simulink model "tvc_sim"  (R2019b)
settings: Solver=FixedStepAuto  StartTime=0.0  StopTime=3  FixedStep=0.001  RelTol=1e-3
values from neighbouring files (symbols this model uses):
  Ft = 300    [dynamics_gui.m]    (also in tvc.m)
  I = 3.5    [dynamics_gui.m]    (also in tvc.m)
  Kd = 60    [dynamics_gui.m]    (also in tvc.m = 5)
  Ki = 0    [dynamics_gui.m]    (also in tvc.m)
  Kp = 20    [dynamics_gui.m]    (also in tvc.m = 40)
  theta_0 = 15    [tvc.m]
  theta_des = 0    [tvc.m]
  theta_max = 30    [tvc.m]
  x_cm = 1.2    [dynamics_gui.m]    (also in tvc.m)
settings Model: Creator=seant  LastModifiedBy=SPak
settings DataIOCC: ReturnWorkspaceOutputs=off
settings DebuggingCC: ArithmeticOperatorsInVariantConditions=warning
settings SFSimCC: SimUseLocalCustomCode=off  CustomCodeUndefinedFunction=UseInterfaceOnly
settings RTWCC: RTWUseLocalCustomCode=off

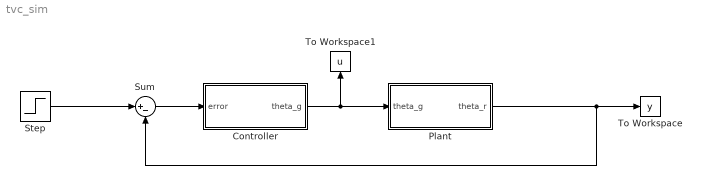
== system tvc_sim ==
  "Controller " : Subsystem
  "Plant " : Subsystem
  Step : Step  Time=0  After=theta_des  SampleTime=0
  Sum : Sum  Inputs=|+-
  To Workspace : ToWorkspace  VariableName=y  SaveFormat=Timeseries  SampleTime=-1
  To Workspace1 : ToWorkspace  VariableName=u  SaveFormat=Timeseries  SampleTime=-1
  wires:
  Step/1 -> Sum/1
  "Controller "/1(theta_g) -> "Plant "/1("theta_g "), To Workspace1/1
  Sum/1 -> "Controller "/1(error)
  "Plant "/1(theta_r) -> Sum/2, To Workspace/1

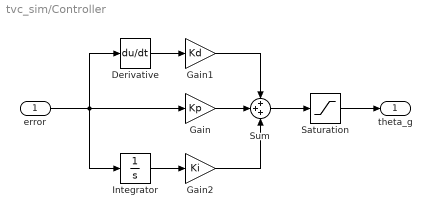
== system tvc_sim/Controller  ==
  error : Inport
  Derivative : Derivative
  Gain : Gain  Gain=Kp
  Gain1 : Gain  Gain=Kd
  Gain2 : Gain  Gain=Ki
  Integrator : Integrator
  Saturation : Saturate  UpperLimit=deg2rad(theta_max)  LowerLimit=-deg2rad(theta_max)
  Sum : Sum  Inputs=+++
  theta_g : Outport  VectorParamsAs1DForOutWhenUnconnected=off
  wires:
  error/1 -> Integrator/1, Derivative/1, Gain/1
  Integrator/1 -> Gain2/1
  Derivative/1 -> Gain1/1
  Sum/1 -> Saturation/1
  Gain/1 -> Sum/2
  Gain1/1 -> Sum/1
  Gain2/1 -> Sum/3
  Saturation/1 -> theta_g/1

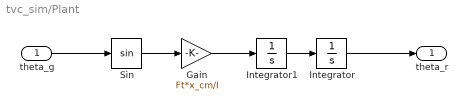
== system tvc_sim/Plant  ==
  "theta_g " : Inport
  Gain : Gain  Gain=Ft*x_cm/I
  Integrator : Integrator  InitialCondition=deg2rad(theta_0)
  Integrator1 : Integrator
  Sin : Trigonometry
  theta_r : Outport  VectorParamsAs1DForOutWhenUnconnected=off
  wires:
  Integrator1/1 -> Integrator/1
  Integrator/1 -> theta_r/1
  "theta_g "/1 -> Sin/1
  Sin/1 -> Gain/1
  Gain/1 -> Integrator1/1
